simulink model "fmcw_range_model"  (R2024b)
settings: Solver=FixedStepDiscrete  StartTime=0.0  StopTime=1.28e-3  FixedStep=5e-9  RelTol=1e-3
undefined symbols (not defined in the file or in its folder): physconst
libraries: phasedenvlib x3, phaseddetectlib x1, phasedwavlib x1
settings Model: Creator=lloyd  LastModifiedBy=lloyd

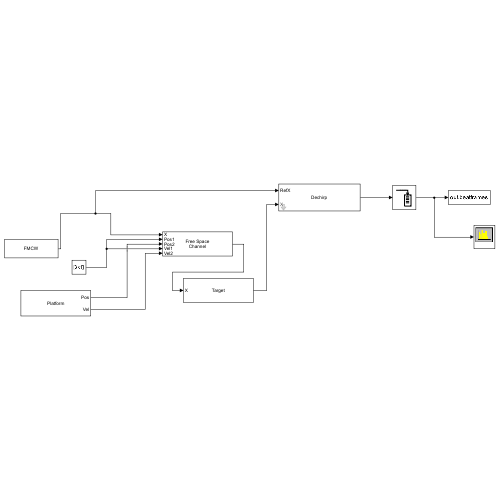
[thumbnail: Simulink's stored preview of the top-level diagram]
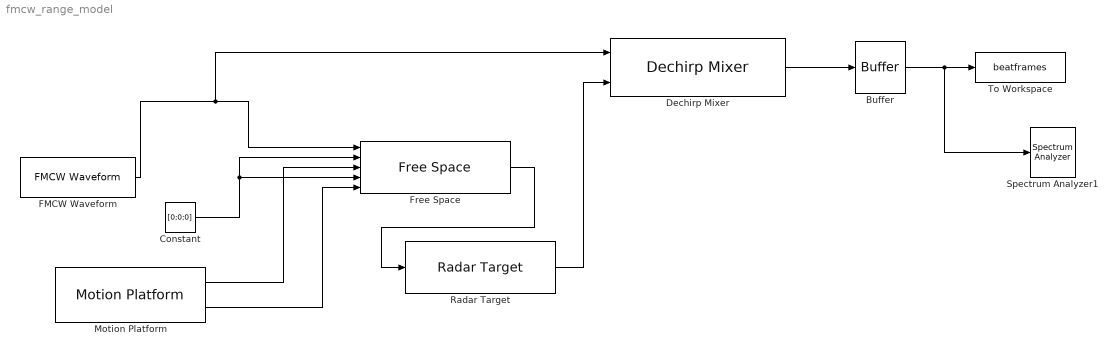
== system fmcw_range_model ==
  Buffer : Buffer  N=2000  OutputFrames=off
  Constant : Constant  Value=[0;0;0]
  Dechirp Mixer : phaseddetectlib/Dechirp Mixer
  FMCW Waveform : phasedwavlib/FMCW Waveform  SampleRate=200e6  SweepTime=10e-6  SweepBandwidth=150e6  SweepDirection=Up  SweepInterval=Positive  OutputFormat=Samples  NumSamples=100  NumSweeps=1  SimulateUsing=Interpreted execution
  Free Space : phasedenvlib/Free Space  PropagationSpeed=3e8  OperatingFrequency=77e9  TwoWayPropagation=on  SampleRateFromInputCheckbox=on  SampleRate=1e6  MaximumDistanceSource=Property  MaximumDistance=500  MaximumNumInputSamplesSource=Auto  MaximumNumInputSamples=1000  SimulateUsing=Interpreted execution
  Motion Platform : phasedenvlib/Motion Platform  MotionModel=Velocity  InitialPosition=[ 50; 0; 0 ]  InitialVelocity=[ 0; 0; 0 ]  VelocitySource=Property  Velocity=[-20;0;0]  AccelerationSource=Property  Acceleration=[0;0;0]  CustomTrajectory=[ 0, 0, 0, 0, 0, 0, 0; 1, 0, 0, 0, 0, 0, 0 ]  ScanMode=None  InitialScanAngle=0  AzimuthSpan=[ -60, 60 ]  AzimuthScanRate=10  InitialOrientationAxes=eye( 3 )  OrientationAxesOutputPort=off  ElapsedTimeSource=Auto  SampleRateFromInputCheckbox=on  SampleRate=1e6  SimulateUsing=Interpreted execution
  Radar Target : phasedenvlib/Radar Target  EnablePolarization=off  Mode=Monostatic  MeanRCSSource=Property  ScatteringMatrixSource=Property  MeanRCS=10  ScatteringMatrix=eye( 2 )  Model=Nonfluctuating  PropagationSpeed=physconst( 'LightSpeed' )  OperatingFrequency=77e9  SeedSource=Auto  Seed=0  SimulateUsing=Interpreted execution
  Spectrum Analyzer1 : SpectrumAnalyzer  WindowPosition=[368.000000,182.000000,800.000000,500.000000,]  ScopeFrameLocation=window  WindowInvariantSamplesPerUpdate=on  Span=200000000.00000003  StartFrequency=-100000000.00000001  StopFrequency=100000000.00000001  YLimits=[-220.96842244868978,-115.55105773868976]  SelectedToolstripTab=spectrumAnalyzerToolstrip.spectrumTab
  To Workspace : ToWorkspace  VariableName=beatframes  SampleTime=-1
  wires:
  FMCW Waveform/1 -> Dechirp Mixer/1, Free Space/1
  Radar Target/1 -> Dechirp Mixer/2
  Free Space/1 -> Radar Target/1
  Dechirp Mixer/1 -> Buffer/1
  Buffer/1 -> To Workspace/1, Spectrum Analyzer1/1
  Motion Platform/1 -> Free Space/3
  Motion Platform/2 -> Free Space/5
  Constant/1 -> Free Space/4, Free Space/2
